simulink library "uavsimBlockset_ServoHS55"  (Simulink 8.4)
settings: Solver=ode45  StartTime=0.0  StopTime=10.0  RelTol=1e-3
settings Model: Creator=mstolle  LastModifiedBy=j.bolting

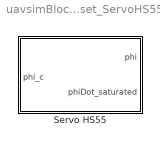
== system uavsimBlockset_ServoHS55 ==
  Servo HS55 : Subsystem  mask{deflectionLimits_rad=[deg2rad(-45) deg2rad(45)], rateLimit_enabled=on, outputLimit_enabled=on, mask_initialPosition=0}
      mask prompts: deflectionLimits_rad "Control surface deflection limits [rad rad]"; rateLimit_enabled "Rate saturation enabled?"; outputLimit_enabled "Output saturation enabled?"; mask_initialPosition "Initial position"

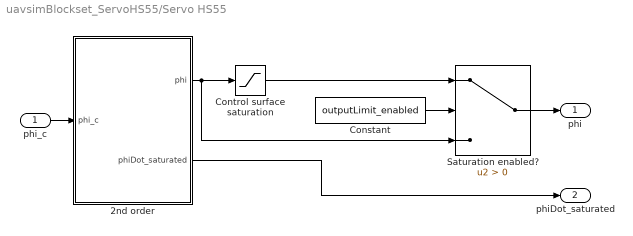
== system uavsimBlockset_ServoHS55/Servo HS55 ==
  phi_c : Inport
  2nd order : Subsystem  mask{wn_fin=10*2*pi, z_fin=0.8, fin_act_0=mask_initialPosition, fin_act_vel=0, rateLimit=deg2rad(60)/0.18}
      mask prompts: wn_fin "Natural frequency"; z_fin "Damping ratio"; fin_act_0 "Initial position"; fin_act_vel "Intial velocity"; rateLimit "Rate limit"
  Constant : Constant  Value=outputLimit_enabled
  Control surface saturation : Saturate  UpperLimit=deflectionLimits_rad(2)  LowerLimit=deflectionLimits_rad(1)
  Saturation enabled? : Switch  Criteria=u2 > Threshold
  phi : Outport  PortDimensions=1
  phiDot_saturated : Outport  Port=2  PortDimensions=1
  wires:
  2nd order/1(phi) -> Control surface saturation/1, Saturation enabled?/3
  Constant/1 -> Saturation enabled?/2
  Saturation enabled?/1 -> phi/1
  2nd order/2(phiDot_saturated) -> phiDot_saturated/1
  Control surface saturation/1 -> Saturation enabled?/1
  phi_c/1 -> 2nd order/1(phi_c)

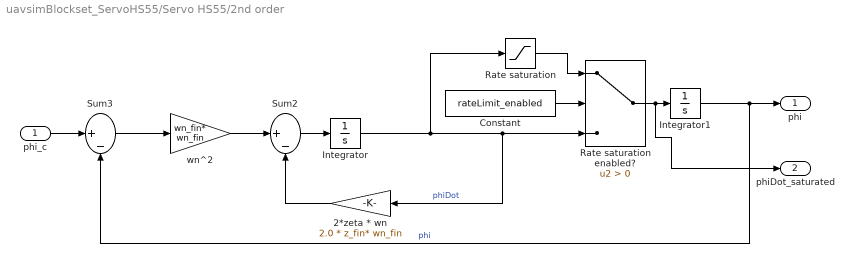
== system uavsimBlockset_ServoHS55/Servo HS55/2nd order ==
  phi_c : Inport
  2*zeta * wn : Gain  Gain=2.0 * z_fin* wn_fin  SaturateOnIntegerOverflow=on  OutDataTypeStr=Inherit: Same as input  ParamDataTypeStr=Inherit: Same as input
  Constant : Constant  Value=rateLimit_enabled
  Integrator : Integrator  InitialCondition=fin_act_vel
  Integrator1 : Integrator  InitialCondition=fin_act_0
  Rate saturation : Saturate  UpperLimit=rateLimit  LowerLimit=-rateLimit
  Rate saturation enabled? : Switch  Criteria=u2 > Threshold
  Sum2 : Sum  Inputs=|+-  SaturateOnIntegerOverflow=on  InputSameDT=on  OutDataTypeStr=Inherit: Same as first input
  Sum3 : Sum  Inputs=|+-  SaturateOnIntegerOverflow=on  InputSameDT=on  OutDataTypeStr=Inherit: Same as first input
  wn^2 : Gain  Gain=wn_fin* wn_fin  SaturateOnIntegerOverflow=on  OutDataTypeStr=Inherit: Same as input  ParamDataTypeStr=Inherit: Same as input
  phi : Outport  PortDimensions=1
  phiDot_saturated : Outport  Port=2  PortDimensions=1
  wires:
  Rate saturation enabled?/1 -> Integrator1/1, phiDot_saturated/1
  Rate saturation/1 -> Rate saturation enabled?/1
  Constant/1 -> Rate saturation enabled?/2
  Integrator/1 -> Rate saturation/1, 2*zeta * wn/1, Rate saturation enabled?/3  "phiDot"
  Sum3/1 -> wn^2/1
  phi_c/1 -> Sum3/1
  2*zeta * wn/1 -> Sum2/2
  Sum2/1 -> Integrator/1
  wn^2/1 -> Sum2/1
  Integrator1/1 -> Sum3/2, phi/1  "phi"
